simulink subsystem "Controllers"  (R2024b)
settings: Solver=VariableStepAuto  StartTime=0.0  StopTime=10.0  RelTol=1e-3
values from neighbouring files (symbols this model uses):
  CarrierFreq = 150    [init_MMC_HVDC_200.m]
  freq_left = 50    [init_MMC_HVDC_200.m]
  freq_right = 50    [init_MMC_HVDC_200.m]
  Ll = 0.04889    [init_MMC_HVDC_200.m]
  nb_cell = numberOfCell    (= 200)    [init_MMC_HVDC_200.m]
  numberOfCell = 200    [init_MMC_HVDC_200.m]
  P_AC = 1000e6    (= 1000000000)    [init_MMC_HVDC_200.m]
  Rl = 0    [init_MMC_HVDC_200.m]
  Tctrl = Ts    (= 3.5e-05)    [init_MMC_HVDC_200.m]
  Ts = 35e-6    (= 3.5e-05)    [init_MMC_HVDC_200.m]
  V_AC_sec = 320e3    (= 320000)    [init_MMC_HVDC_200.m]
undefined symbols (not defined in the file or in its folder): dend, DiscIntNeverNeededParam, numd
libraries: powerlib_extras x12, simulink x10
(part 1 of 4)
Description:
  | MMC HVDC controllers
settings Model: Creator=Kyle  LastModifiedBy=CD8435

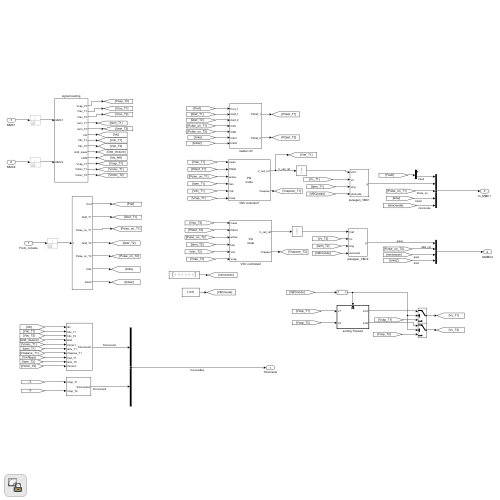
[thumbnail: Simulink's stored preview of the top-level diagram]
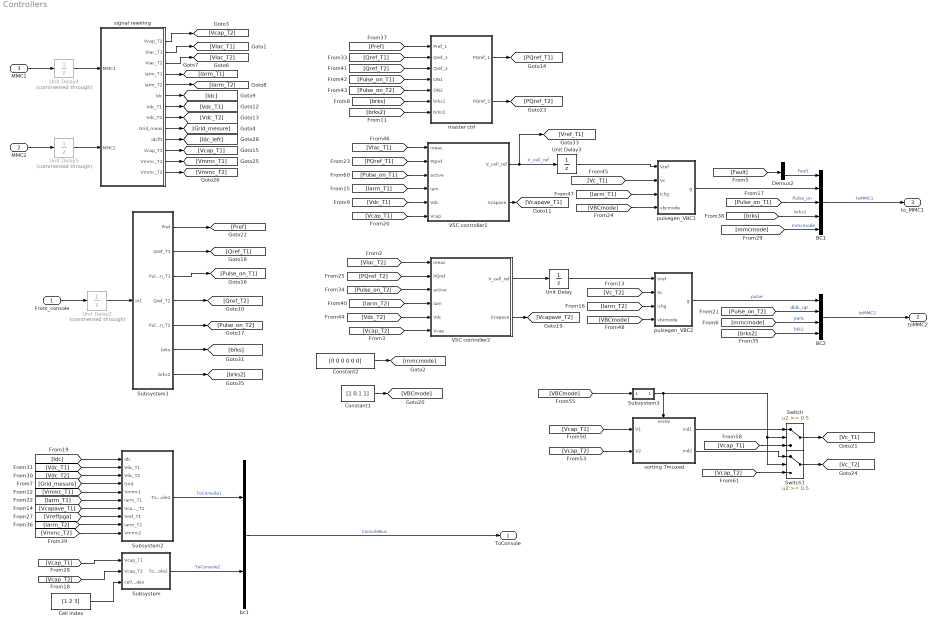
== system Controllers ==
  From_console : Inport
  MMC2 : Inport  Port=2
  MMC1 : Inport  Port=3
  BC1 : BusCreator  Inputs=5  OutDataTypeStr=Bus: toMMC1  NonVirtualBus=on
  BC2 : BusCreator  Inputs=4  OutDataTypeStr=Bus: toMMC2  NonVirtualBus=on
  Cell index : Constant  Value=[1 2 3]
  Constant1 : Constant  Value=[1 0.1 1]
  Constant2 : Constant  Value=[0 0 0 0 0 0]
  Demux2 : Demux  Outputs=2
  Subsystem : Subsystem
  Subsystem1 : Subsystem  mask{brk1=0.15, brk2=0.15, act1=0.25, act2=0.25}
  Subsystem2 : Subsystem
  Subsystem3 : Subsystem
  Switch : Switch  Threshold=0.5  SaturateOnIntegerOverflow=off  InputSameDT=off
  Switch1 : Switch  Threshold=0.5  SaturateOnIntegerOverflow=off  InputSameDT=off
  Unit Delay : UnitDelay  SampleTime=Ts  HasFrameUpgradeWarning=on
  Unit Delay2 : UnitDelay  Commented=through  SampleTime=Ts  HasFrameUpgradeWarning=on
  Unit Delay3 : UnitDelay  SampleTime=Ts  HasFrameUpgradeWarning=on
  Unit Delay4 : UnitDelay  Commented=through  SampleTime=Ts  HasFrameUpgradeWarning=on
  Unit Delay5 : UnitDelay  Commented=through  SampleTime=Ts  HasFrameUpgradeWarning=on
  VSC controller1 : Subsystem  mask(MMC converter controller){cm=off, base=[P_AC, V_AC_sec*1,  E, freq_left], LRx=[Ll, Rl]/2, LRx_inpu=off, Kd=[0.3  2]*10/6  %was [1 0.1]   ; [0.1  1]*1, Kp=[0.3 1]*1     %was [1 0.1]   ; [0.1  1]*1, Kvdc=[0.5*4*1 0.5*2]*1;   %was [0.5 1]*20 for Cdc=320uF, Vabc_lim=[-1 1], limitVdq=1.1, nadv=6, xtrIctrl1=[0.4 10 10 -10], Ts=Tctrl}
      mask prompts: cm "Control mode (check VQ/uncheck PQ), only one terminal in VQ mode"; base "Base value for power(VA), ac voltage(V), dc voltage to ground(V), and frequenvy(Hz) [Sb, Vb, Vdcb,freq]"; LRx "commutation inductance and resistance [Lx, Rx]"; LRx_inpu "[Lx, Rx] in pu if checked/ SI unchecked"; Kd "Kp Ki for d-axis PI control [kp ki]"; Kp "Kp Ki for q-axis PI control [kp ki]"; Kvdc "Kp Ki for Vdc PI control [kp ki]"; Vabc_lim "output Vabc limit [min max]"; limitVdq "Limit for Vd,Vq (pu, default = 1.1)"; nadv "nb of time step to compesate for delay (default=1)"; xtrIctrl1 "[kp, kp, limitmax, limitmin] for current control (default=[0.4, 10, 10, -10])"
      mask init:
      | if cm==0;
      |     x=['PQ\nmode'];
      | else
      |     x=['VQ\nmode'];
      | end
      | 
      | Sb=base(1);            %VA 3phase power base;
      | Vb=base(2);       %V, line-line rms voltage base
      | Ib=Sb/(sqrt(3)*Vb); %A, rms current base
      | Zb=Vb^2/Sb ;        %ohm, impedence base
      | Vdc=base(3);      %V Vdc+ to ground or ground to Vdc- 
      | frq=base(4);
      | 
      | if LRx_inpu
      |     Rxpu=LRx(2);
      |     Lxpu=LRx(1);
      | else
      |     Rxpu=LRx(2)/Zb;
      |     Lxpu=LRx(1)*2*pi*frq/Zb;
      | end;
      | 
      | ks=Vdc*sqrt(3/2)/Vb;     % ma=1/ks for 1pu dc ->1pu ac;
      | 
      | Kp=Kd;
      mask DialogControl ParameterTabVar0 Prompt: Parameters
      mask DialogControl ParameterTabVar01 Prompt: Advanced
      mask Display: disp (x);
  VSC controller2 : Subsystem  mask(MMC converter controller){cm=on, base=[P_AC, V_AC_sec*1,  E, freq_right], LRx=[Ll, Rl]/2, LRx_inpu=off, Kd=[0.3  2]*10/6  %was [1 0.1]   ; [0.1  1]*1, Kp=[0.3 1]*1     %was [1 0.1]   ; [0.1  1]*1, Kvdc=[0.5*4*1 0.5*2]*1;   %was [0.5 1]*20 for Cdc=320uF, Vabc_lim=[-1 1], limitVdq=1.1, nadv=6, xtrIctrl1=[0.4 10 10 -10], Ts=Tctrl}
      mask prompts: cm "Control mode (check VQ/uncheck PQ), only one terminal in VQ mode"; base "Base value for power(VA), ac voltage(V), dc voltage to ground(V), and frequenvy(Hz) [Sb, Vb, Vdcb,freq]"; LRx "commutation inductance and resistance [Lx, Rx]"; LRx_inpu "[Lx, Rx] in pu if checked/ SI unchecked"; Kd "Kp Ki for d-axis PI control [kp ki]"; Kp "Kp Ki for q-axis PI control [kp ki]"; Kvdc "Kp Ki for Vdc PI control [kp ki]"; Vabc_lim "output Vabc limit [min max]"; limitVdq "Limit for Vd,Vq (pu, default = 1.1)"; nadv "nb of time step to compesate for delay (default=1)"; xtrIctrl1 "[kp, kp, limitmax, limitmin] for current control (default=[0.4, 10, 10, -10])"
      mask init: same as Controllers/VSC controller1
      mask DialogControl ParameterTabVar0 Prompt: Parameters
      mask DialogControl ParameterTabVar01 Prompt: Advanced
      mask Display: disp (x);
  bc1 : BusCreator  Inputs=2  OutDataTypeStr=Bus: ConsoleBus  NonVirtualBus=on
  master ctrl : Subsystem
  pulsegen_VBC1 : Subsystem
  pulsegen_VBC2 : Subsystem
  signal rewiring : Subsystem
  sorting Tmuxed : Subsystem
  ToConsole : Outport  VectorParamsAs1DForOutWhenUnconnected=off
  toMMC2 : Outport  Port=2  VectorParamsAs1DForOutWhenUnconnected=off
  to_MMC1 : Outport  Port=3  VectorParamsAs1DForOutWhenUnconnected=off
  wires:
  Subsystem2/1(ToConsole1) -> bc1/1  "ToConsole1"
  From_console/1 -> Unit Delay2/1
  MMC1/1 -> Unit Delay4/1
  MMC2/1 -> Unit Delay5/1
  Subsystem/1(ToConsole2) -> bc1/2  "ToConsole2"
  [Idc] -> Subsystem2/1(Idc)
  [Vdc_T1] -> Subsystem2/2(Vdc_T1)
  [Vdc_T2] -> Subsystem2/3(Vdc_T2)
  [Grid_mesure] -> Subsystem2/4(Grid)
  [Vmmc_T1] -> Subsystem2/5(Vmmc1)
  [Iarm_T1] -> Subsystem2/6(Iarm_T1)
  [Vcapave_T1] -> Subsystem2/7(Vcapave_T1)
  [Vreffpga] -> Subsystem2/8(Vref_T1)
  [Iarm_T2] -> Subsystem2/9(Iarm_T2)
  [Vmmc_T2] -> Subsystem2/10(Vmmc2)
  [Vcap_T1] -> Subsystem/1(Vcap_T1)
  [Vcap_T2] -> Subsystem/2(Vcap_T2)
  signal rewiring/1(Vcap_T2) -> [Vcap_T2]
  signal rewiring/2(VIac_T1) -> [VIac_T1]
  signal rewiring/3(VIac_T2) -> [VIac_T2]
  signal rewiring/4(Iarm_T1) -> [Iarm_T1]
  signal rewiring/5(Iarm_T2) -> [Iarm_T2]
  signal rewiring/9(Grid_meas) -> [Grid_mesure]
  signal rewiring/6(Idc) -> [Idc]
  signal rewiring/7(Vdc_T1) -> [Vdc_T1]
  signal rewiring/8(Vdc_T2) -> [Vdc_T2]
  signal rewiring/10(Idcflt) -> [Idc_left]
  signal rewiring/11(Vcap_T1) -> [Vcap_T1]
  signal rewiring/12(Vmmc_T1) -> [Vmmc_T1]
  signal rewiring/13(Vmmc_T2) -> [Vmmc_T2]
  Subsystem1/2(Qref_T1) -> [Qref_T1]
  Subsystem1/4(Qref_T2) -> [Qref_T2]
  Subsystem1/1(Pref) -> [Pref]
  Subsystem1/6(brks) -> [brks]
  Subsystem1/7(brks2) -> [brks2]
  Subsystem1/5(Pulse_on_T2) -> [Pulse_on_T2]
  Subsystem1/3(Pulse_on_T1) -> [Pulse_on_T1]
  [Vcap_T1] -> sorting Tmuxed/1(V1)
  [Vcap_T2] -> sorting Tmuxed/2(V2)
  sorting Tmuxed/1(ind1) -> Switch/1
  sorting Tmuxed/2(ind2) -> Switch1/1
  [VBCmode] -> Subsystem3/1(In1)
  Subsystem3/1(Out1) -> sorting Tmuxed/Enable, Switch/2, Switch1/2
  Switch/1 -> [Vc_T1]
  [Vcap_T1] -> Switch/3
  Switch1/1 -> [Vc_T2]
  [Vcap_T2] -> Switch1/3
  [Fault] -> Demux2/1
  VSC controller2/1(V_cell_ref) -> Unit Delay/1
  [Pref] -> master ctrl/1(Pref_1)
  [Qref_T1] -> master ctrl/2(Qref_1)
  [Qref_T2] -> master ctrl/3(Qref_2)
  master ctrl/1(PQref_1) -> [PQref_T1]
  master ctrl/2(PQref_2) -> [PQref_T2]
  [Pulse_on_T1] -> master ctrl/4(ON1)
  [Pulse_on_T2] -> master ctrl/5(ON2)
  [Pulse_on_T1] -> VSC controller1/3(active)
  [VIac_T1] -> VSC controller1/1(meas)
  [PQref_T1] -> VSC controller1/2(PQref)
  [Iarm_T1] -> VSC controller1/4(Iam)
  VSC controller1/1(V_cell_ref) -> [Vref_T1], Unit Delay3/1  "V_cell_ref"
  [Pulse_on_T2] -> BC2/2  "dblk_rgt"
  [mmcmode] -> BC2/3  "para"
  [brks2] -> BC2/4  "brk2"
  [Vdc_T1] -> VSC controller1/5(Vdc)
  [Vcap_T1] -> VSC controller1/6(Vcap)
  VSC controller1/2(Vcapave) -> [Vcapave_T1]
  [VIac_T2] -> VSC controller2/1(meas)
  [PQref_T2] -> VSC controller2/2(PQref)
  [Pulse_on_T2] -> VSC controller2/3(active)
  [Iarm_T2] -> VSC controller2/4(Iam)
  [Vdc_T2] -> VSC controller2/5(Vdc)
  [Vcap_T2] -> VSC controller2/6(Vcap)
  VSC controller2/2(Vcapave) -> [Vcapave_T2]
  [brks] -> master ctrl/6(brks1)
  [brks2] -> master ctrl/7(brks2)
  pulsegen_VBC2/1(g) -> BC2/1  "pulse"
  [Pulse_on_T1] -> BC1/3  "Pulse_on"
  [brks] -> BC1/4  "brks2"
  Demux2/2 -> BC1/1  "Fault"
  [mmcmode] -> BC1/5  "mmcmode"
  [Vc_T1] -> pulsegen_VBC1/2(Vc)
  [Iarm_T1] -> pulsegen_VBC1/3(ichg)
  pulsegen_VBC1/1(g) -> BC1/2
  [VBCmode] -> pulsegen_VBC1/4(vbcmode)
  [Vc_T2] -> pulsegen_VBC2/2(Vc)
  [Iarm_T2] -> pulsegen_VBC2/3(ichg)
  [VBCmode] -> pulsegen_VBC2/4(vbcmode)
  Constant1/1 -> [VBCmode]
  Constant2/1 -> [mmcmode]
  Unit Delay/1 -> pulsegen_VBC2/1(Vref)
  Unit Delay3/1 -> pulsegen_VBC1/1(Vref)
  Unit Delay4/1 -> signal rewiring/1(MMC1)
  Unit Delay5/1 -> signal rewiring/2(MMC2)
  Unit Delay2/1 -> Subsystem1/1(In1)
  BC1/1 -> to_MMC1/1  "toMMC1"
  BC2/1 -> toMMC2/1  "toMMC2"
  bc1/1 -> ToConsole/1  "ConsoleBus"
  Cell index/1 -> Subsystem/3(cellindex)

== system Controllers/Subsystem ==
  Vcap_T1 : Inport
  Vcap_T2 : Inport  Port=2
  cellindex : Inport  Port=3
  Bus Creator : BusCreator  Inputs=2
  Subsystem1 : Subsystem
  Subsystem3 : Subsystem
  ToConsole2 : Outport  VectorParamsAs1DForOutWhenUnconnected=off
  wires:
  cellindex/1 -> Subsystem1/2(CellIndex)
  Vcap_T2/1 -> Subsystem3/1(In1)
  Vcap_T1/1 -> Subsystem1/1(In1)
  Bus Creator/1 -> ToConsole2/1
  Subsystem1/1(Out1) -> Bus Creator/1  "Vcap_T1"
  Subsystem3/1(Out1) -> Bus Creator/2  "Vcap_T2"

== system Controllers/Subsystem1 ==
  In1 : Inport
  Bus Selector : BusSelector  OutputSignals=PQref.Pref,PQref.Qref_T1,PQref.Pulse_on_T1,Q2.signal1,Q2.Pulse_on_T2,breakers.dcbrk,breakers.ac_brk_T1,breakers.ac_brk_T2
  Mux5 : Mux  Inputs=2
  Product{,1..3} (4 alike) : Product  RndMeth=Zero
  Step : Step  Time=brk1  SampleTime=Ts
  Step1 : Step  Time=brk2  SampleTime=Ts
  Step2 : Step  Time=act2  SampleTime=Ts
  Step3 : Step  Time=act1  SampleTime=Ts
  Pref : Outport  VectorParamsAs1DForOutWhenUnconnected=off
  Qref_T1 : Outport  Port=2  VectorParamsAs1DForOutWhenUnconnected=off
  Pulse_on_T1 : Outport  Port=3  VectorParamsAs1DForOutWhenUnconnected=off
  Qref_T2 : Outport  Port=4  VectorParamsAs1DForOutWhenUnconnected=off
  Pulse_on_T2 : Outport  Port=5  VectorParamsAs1DForOutWhenUnconnected=off
  brks : Outport  Port=6  VectorParamsAs1DForOutWhenUnconnected=off
  brks2 : Outport  Port=7  VectorParamsAs1DForOutWhenUnconnected=off
  wires:
  Step/1 -> Product/2
  Step1/1 -> Product1/2
  Step2/1 -> Product2/2
  Bus Selector/5 -> Product2/1  "<Pulse_on_T2>"
  Bus Selector/3 -> Product3/1  "<Pulse_on_T1>"
  Step3/1 -> Product3/2
  Bus Selector/2 -> Qref_T1/1  "<Qref_T1>"
  Product3/1 -> Pulse_on_T1/1
  Bus Selector/4 -> Qref_T2/1  "<signal1>"
  In1/1 -> Bus Selector/1
  Product2/1 -> Pulse_on_T2/1
  Product/1 -> brks/1
  Product1/1 -> brks2/1
  Mux5/1 -> Product/1
  Bus Selector/1 -> Pref/1  "<Pref>"
  Bus Selector/6 -> Mux5/1  "<dcbrk>"
  Bus Selector/7 -> Mux5/2  "<ac_brk_T1>"
  Bus Selector/8 -> Product1/1  "<ac_brk_T2>"

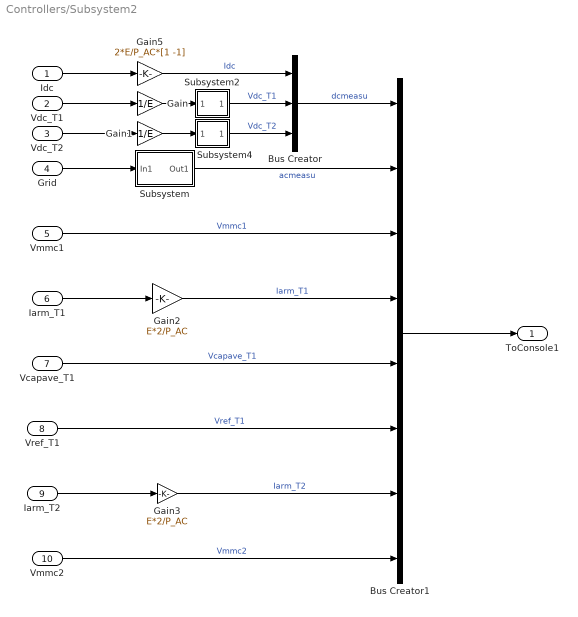
== system Controllers/Subsystem2 ==
  Idc : Inport
  Vdc_T1 : Inport  Port=2
  Vdc_T2 : Inport  Port=3
  Grid : Inport  Port=4
  Vmmc1 : Inport  Port=5
  Iarm_T1 : Inport  Port=6
  Vcapave_T1 : Inport  Port=7
  Vref_T1 : Inport  Port=8
  Iarm_T2 : Inport  Port=9
  Vmmc2 : Inport  Port=10
  Bus Creator : BusCreator  Inputs=3
  Bus Creator1 : BusCreator  Inputs=8
  Gain : Gain  Gain=1/E
  Gain1 : Gain  Gain=1/E
  Gain2 : Gain  Gain=E*2/P_AC
  Gain3 : Gain  Gain=E*2/P_AC
  Gain5 : Gain  Gain=2*E/P_AC*[1 -1]
  Subsystem : Subsystem
  Subsystem2 : Subsystem
  Subsystem4 : Subsystem
  ToConsole1 : Outport  VectorParamsAs1DForOutWhenUnconnected=off
  wires:
  Subsystem4/1(Out1) -> Bus Creator/3  "Vdc_T2"
  Subsystem2/1(Out1) -> Bus Creator/2  "Vdc_T1"
  Gain3/1 -> Bus Creator1/7  "Iarm_T2"
  Iarm_T2/1 -> Gain3/1
  Vmmc2/1 -> Bus Creator1/8  "Vmmc2"
  Vref_T1/1 -> Bus Creator1/6  "Vref_T1"
  Vcapave_T1/1 -> Bus Creator1/5  "Vcapave_T1"
  Vmmc1/1 -> Bus Creator1/3  "Vmmc1"
  Iarm_T1/1 -> Gain2/1
  Vdc_T2/1 -> Gain1/1
  Vdc_T1/1 -> Gain/1
  Grid/1 -> Subsystem/1(In1)
  Bus Creator1/1 -> ToConsole1/1
  Gain2/1 -> Bus Creator1/4  "Iarm_T1"
  Subsystem/1(Out1) -> Bus Creator1/2  "acmeasu"
  Gain1/1 -> Subsystem4/1(In1)
  Gain/1 -> Subsystem2/1(In1)
  Gain5/1 -> Bus Creator/1  "Idc"
  Idc/1 -> Gain5/1
  Bus Creator/1 -> Bus Creator1/1  "dcmeasu"

== system Controllers/Subsystem3 ==
  In1 : Inport
  Compare To Constant1 : simulink/Logic and Bit Operations/Compare To Constant  relop===  const=2  OutDataTypeStr=uint8
  Compare To Constant2 : simulink/Logic and Bit Operations/Compare To Constant  relop===  const=12  OutDataTypeStr=uint8
  Demux1 : Demux  Outputs=[1 -1]
  Logical Operator : Logic  Operator=OR  AllPortsSameDT=off  OutDataTypeStr=boolean
  Out1 : Outport  VectorParamsAs1DForOutWhenUnconnected=off
  wires:
  Logical Operator/1 -> Out1/1
  Demux1/1 -> Compare To Constant1/1, Compare To Constant2/1
  Compare To Constant2/1 -> Logical Operator/2
  Compare To Constant1/1 -> Logical Operator/1
  In1/1 -> Demux1/1

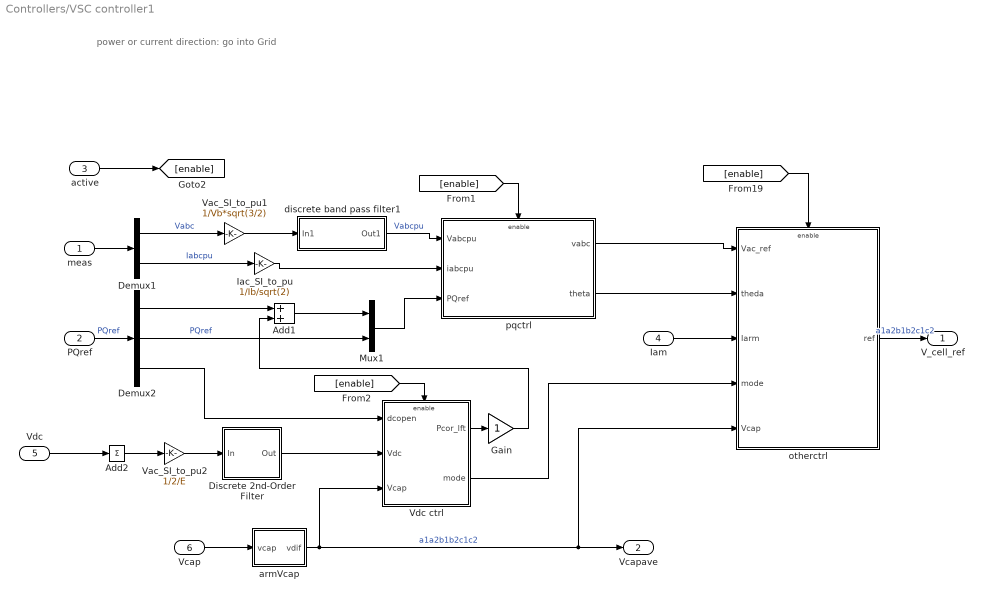
== system Controllers/VSC controller1 ==
  note: power or current direction: go into Grid
  meas : Inport
  PQref : Inport  Port=2
  active : Inport  Port=3
  Iam : Inport  Port=4
  Vdc : Inport  Port=5
  Vcap : Inport  Port=6
  Add1 : Sum
  Add2 : Sum  Inputs=1
  Demux1 : Demux  Outputs=[3 3 ]
  Demux2 : Demux  Outputs=3
  Discrete 2nd-Order Filter : Subsystem  mask(Discrete 2nd-Order Filter){FilterType=Lowpass, Fo=90, Zeta=0.707, Ts=Ts, Initialize=off, Vac_Init=[0.8 -25 60], Vdc_Init=-0.4, PlotResponse=off, param1=[1 500 1]}
      mask prompts: FilterType "Filter Type:"; Fo "Cut-off frequency (Hz):"; Zeta "Damping factor Zeta ( Q = 1 / (2*Zeta) ):"; Ts "Sample time:"; Initialize "Initialize filter states"; Vac_Init "AC initial input: [ Mag  Phase(degrees)  Freq(Hz) ]"; Vdc_Init "DC Initial input:"; PlotResponse "Plot filter response"; param1 "Frequency range(Hz) : [Start  End  Inc.]"
      mask init:
      | str=sprintf(' Fo=%iHz\n\n',Fo);
      | Wo=2*pi*Fo;
      | switch FilterType
      | case 1, % Lowpass
      |        X=[0 1 2 3 4];
      |        Y=[-2 -2 -3 -4 -4];
      |        n2=0;n1=0;n0=Wo*Wo;
      |        d2=1;d1=2*Zeta*Wo;d0=Wo*Wo;
      | 	   Ystep=1;
      |  case 2,   % Highpass
      |        X=[0 1 2 3 4];
      |        Y=[-4 -4 -3 -2 -2];
      |        n2=1;n1=0;n0=0;
      |        d2=1;d1=2*Zeta*Wo;d0=Wo*Wo;
      | 	   Ystep=2;
      |     case 3,   % Bandpass
      |        X=[0 1 2 3 4 5 ];
      |        Y=[-3 -3 -2 -2 -3 -3];
      |        n2=0;n1=2*Zeta*Wo;n0=0;
      |        d2=1;d1=2*Zeta*Wo;d0=Wo*Wo;
      | 	   Ystep=3;
      |     case 4,  %Bandstop (Notch)
      |        X=[0 1 2 3 4 5 ];
      |        Y=[-2 -2 -3 -3 -2 -2];
      |        n2=1;n1=0;n0=Wo*Wo;
      |        d2=1;d1=2*Zeta*Wo;d0=Wo*Wo;
      | 	   Ystep=4;
      |     end
      | %
      | numc=[n2 n1 n0];
      | denc=[d2 d1 d0];
      | [Ac,Bc,Cc,Dc]=tf2ss(numc,denc);
      | %
      | %  Conversion to discrete transfer function
      | nstates = size(Ac,1);
      | invexp = inv(eye(nstates) - (Ts/2)*Ac);
      | Ad = invexp*(eye(nstates) + (Ts/2)*Ac);
      | Bd = invexp*Bc;
      | Cd = Cc*invexp*Ts;
      | Dd = Cc*invexp*Bc*(Ts/2) + Dc;
      | %
      | if Initialize==1  % Compute initial conditions on states
      | u1=Vac_Init(1)*exp(j*Vac_Init(2)*pi/180);
      | u2=Vdc_Init*exp(j*90*pi/180);
      | u=u1+u2;
      | u0=imag(u); % input at  t=0;
      | I=eye(size(Ac));
      | sI1=I*j*(2*pi*Vac_Init(3));
      | sI2=I*j*0;
      | x=inv(sI1-Ac)*Bc*u1 + inv(sI2-Ac)*Bc*u2;
      | x0c=imag(x);
      | x0d=(I-Ac*Ts/2)*x0c/Ts - Bc/2*u0;
      | else
      | x0d=0;
      | end
      | %
      | if PlotResponse==1 % Plot frequency and step response
      | if Zeta==1
      | 	z=1+1e-12;
      | else
      | 	z=Zeta;
      | end
      | wn=Wo;
      | t=[0:1/(z*wn)/1000:7/(z*wn)];
      | f=param1(1):param1(3):param1(2);
      | w=2*pi*f;
      | switch FilterType
      | 	case 1, % Lowpass
      | 		Ystep=wn^2*(1/wn^2+1/(4*z^2*wn^2-4*wn^2)^(1/2)*(1/(-z*wn+1/2*(4*z^2*wn^2-4*wn^2)^(1/2))*exp((-z*wn+1/2*(4*z^2*wn^2-4*wn^2)^(1/2))*t)-1/(-z*wn-1/2*(4*z^2*wn^2-4*wn^2)^(1/2))*exp((-z*wn-1/2*(4*z^2*wn^2-4*wn^2)^(1/2))*t)));
      | 		numFreq=wn^2;
      | 	case 2,   % Highpass
      | 		Ystep=-exp(-z*wn*t)/(z-1)/(z+1).*cos((-wn^2*(z-1)*(z+1))^(1/2)*t)+exp(-z*wn*t)/(z-1)/(z+1)*z^2.*cos((-wn^2*(z-1)*(z+1))^(1/2)*t)+z/wn*exp(-z*wn*t)/(z-1)/(z+1)*(wn^2-z^2*wn^2)^(1/2).*sin((-wn^2*(z-1)*(z+1))^(1/2)*t);
      | 		numFreq=-w.^2;
      | 	case 3,   % Bandpass
      | 		Ystep=2*z*wn/(4*z^2*wn^2-4*wn^2)^(1/2)*(exp((-z*wn+1/2*(4*z^2*wn^2-4*wn^2)^(1/2))*t)-exp((-z*wn-1/2*(4*z^2*wn^2-4*wn^2)^(1/2))*t));
      | 		numFreq=2*Zeta*wn.*w*j;
      | 	case 4,  %Bandstop (Notch)
      | 		Ystep=1+2*z/wn*exp(-z*wn*t)/(z-1)/(z+1)*(wn^2-z^2*wn^2)^(1/2).*sin((-wn^2*(z-1)*(z+1))^(1/2)*t);	
      | 		numFreq=wn^2-w.^2;
      | end
      | %
      | denFreq=(wn^2-w.^2) + 2*Zeta*wn*j.*w;
      | RepFreq=numFreq./denFreq;
      | Mag=abs(RepFreq);
      | Pha=angle(RepFreq)*180/pi;
      | %
      | figure(1)
      | subplot(2,1,1)
      | plot(f,Mag)
      | grid
      | title('Bode Diagram')
      | ylabel('Magnitude')
      | subplot(2,1,2)
      | plot(f,Pha)
      | ylabel('Phase (deg)')
      | xlabel('Frequency (Hz)')
      | grid
      | figure(2)
      | plot(t,real(Ystep))
      | grid
      | ylabel('Amplitude')
      | xlabel('Time (s)')
      | title('Step Response')
      | end
      | power_initmask();
      mask Help: This block is part of a subset of blocks in the Extras library that does not have documentation associated with it, other than the block mask description.
      mask TypeOptions FilterType: Lowpass | Highpass | Bandpass | Bandstop (Notch)
      mask Callback Initialize: p5=get_param(gcb,'Initialize');if strcmp(p5,'on');visible={'on','on','on','on','on','on','on','on',get_param(gcb,'PlotResponse')};else;visible={'on','on','on','on','on','off','off','on',get_param(gcb,'PlotResponse')};end;set_param(gcb,'MaskVisibilities',visible)
      mask Callback PlotResponse: p8=get_param(gcb,'PlotResponse');if strcmp(p8,'on');visible={'on','on','on','on','on',get_param(gcb,'Initialize'),get_param(gcb,'Initialize'),'on','on'};else;visible={'on','on','on','on','on',get_param(gcb,'Initialize'),get_param(gcb,'Initialize'),'on','off'};end;set_param(gcb,'MaskVisibilities',visible)
      mask Display:
      | plot(X,Y);
      | disp(str);
  Gain : Gain
  Iac_SI_to_pu : Gain  Gain=1/Ib/sqrt(2)
  Mux1 : Mux  Inputs=2
  Vac_SI_to_pu1 : Gain  Gain=1/Vb*sqrt(3/2)
  Vac_SI_to_pu2 : Gain  Gain=1/2/E  SampleTime=Tctrl
  Vdc ctrl : Subsystem
  armVcap : Subsystem
  discrete band pass filter1 : Subsystem  mask(discrete transfer Fcn generator){Fo=frq, adj1=1, inistate=0, Ts=Ts, bodedw=off}
      mask prompts: Fo "F0 (Hz)"; adj1 "adj (1 for no adjustment, larger adj for wider band pass)"; inistate "Initial states"; Ts "Sample time (must be explicite)"; bodedw "draw Bode diagram of filter"
      mask help:
      | This block transfer a continous TF to a discrete TF
      | using Bilinear (Tustin) approximation
      mask init:
      | AD1=tf([1 0],1);
      | 
      | %second order
      | % Fo=50; %cut off freq.
      | % omega0=Fo*2*pi;
      | % adj1=3;   %adjustment 1
      | Zeta= 0.707*adj1; %Damping factor Zeta ( Q = 1 / (2*Zeta) ):
      | Wo=2*pi*Fo;
      | % str=sprintf(' Fo=%iHz\n\n',Fo);
      |  n2=0; n1=0;n0=Wo*Wo;
      |  d2=1;d1=2*Zeta*Wo;d0=Wo*Wo;
      | numc=[n2 n1 n0];
      | denc=[d2 d1 d0];
      | AD3=tf(numc,denc);
      | 
      | AD4=AD1*AD3;
      | [mag1,pha1]=bode(AD4,Wo);
      | mag0=mag1;
      | AD=AD4/mag0;
      | 
      | if bodedw==1
      |     figure;
      |     h=bodeplot(AD1,AD3,AD);
      |     setoptions(h,'FreqUnits','Hz');
      |     grid on;
      |     title(['Bode Diagram, adj=',num2str(adj1)]);
      | end;
      |     
      | % gg=tf(num,den);
      | ggd=c2d(AD,Ts,'tustin');
      | [numd,dend] = tfdata(ggd,'v');
  otherctrl : Subsystem
  pqctrl : Subsystem
  V_cell_ref : Outport  VectorParamsAs1DForOutWhenUnconnected=off
  Vcapave : Outport  Port=2  VectorParamsAs1DForOutWhenUnconnected=off
  wires:
  otherctrl/1(ref) -> V_cell_ref/1  "a1a2b1b2c1c2"
  pqctrl/2(theta) -> otherctrl/2(theda)
  pqctrl/1(vabc) -> otherctrl/1(Vac_ref)
  PQref/1 -> Demux2/1  "PQref"
  active/1 -> [enable]
  Iam/1 -> otherctrl/3(Iarm)
  discrete band pass filter1/1(Out1) -> pqctrl/1(Vabcpu)  "Vabcpu"
  meas/1 -> Demux1/1
  Demux1/2 -> Iac_SI_to_pu/1  "Iabcpu"
  Demux1/1 -> Vac_SI_to_pu1/1  "Vabc"
  Iac_SI_to_pu/1 -> pqctrl/2(iabcpu)
  Vdc/1 -> Add2/1
  Vcap/1 -> armVcap/1(vcap)
  armVcap/1(vdif) -> Vdc ctrl/3(Vcap), Vcapave/1, otherctrl/5(Vcap)  "a1a2b1b2c1c2"
  Vdc ctrl/2(mode) -> otherctrl/4(mode)
  Demux2/1 -> Add1/1
  Vdc ctrl/1(Pcor_lft) -> Gain/1
  Add1/1 -> Mux1/1
  Demux2/2 -> Mux1/2  "PQref"
  Mux1/1 -> pqctrl/3(PQref)
  Discrete 2nd-Order Filter/1(Out) -> Vdc ctrl/2(Vdc)
  Add2/1 -> Vac_SI_to_pu2/1
  Vac_SI_to_pu2/1 -> Discrete 2nd-Order Filter/1(In)
  Gain/1 -> Add1/2
  Vac_SI_to_pu1/1 -> discrete band pass filter1/1(In1)
  Demux2/3 -> Vdc ctrl/1(dcopen)
  [enable] -> otherctrl/Enable
  [enable] -> pqctrl/Enable
  [enable] -> Vdc ctrl/Enable

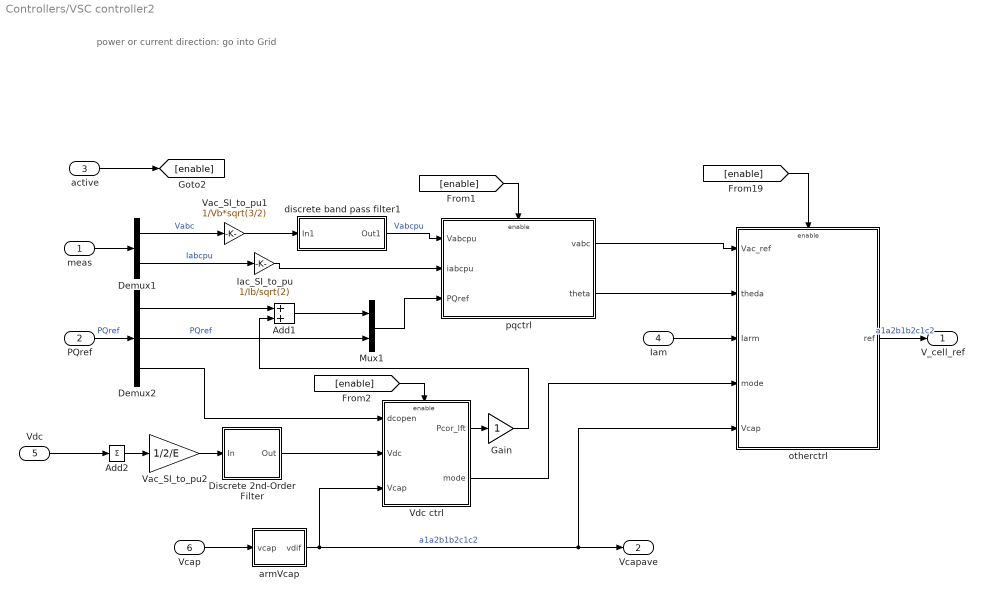
== system Controllers/VSC controller2 ==
  note: power or current direction: go into Grid
  meas : Inport
  PQref : Inport  Port=2
  active : Inport  Port=3
  Iam : Inport  Port=4
  Vdc : Inport  Port=5
  Vcap : Inport  Port=6
  Add1 : Sum
  Add2 : Sum  Inputs=1
  Demux1 : Demux  Outputs=[3 3 ]
  Demux2 : Demux  Outputs=3
  Discrete 2nd-Order Filter : Subsystem  mask(Discrete 2nd-Order Filter){FilterType=Lowpass, Fo=90, Zeta=0.707, Ts=Ts, Initialize=off, Vac_Init=[0.8 -25 60], Vdc_Init=-0.4, PlotResponse=off, param1=[1 500 1]}
      mask prompts: FilterType "Filter Type:"; Fo "Cut-off frequency (Hz):"; Zeta "Damping factor Zeta ( Q = 1 / (2*Zeta) ):"; Ts "Sample time:"; Initialize "Initialize filter states"; Vac_Init "AC initial input: [ Mag  Phase(degrees)  Freq(Hz) ]"; Vdc_Init "DC Initial input:"; PlotResponse "Plot filter response"; param1 "Frequency range(Hz) : [Start  End  Inc.]"
      mask init: same as Controllers/VSC controller1/Discrete 2nd-Order Filter
      mask Help: This block is part of a subset of blocks in the Extras library that does not have documentation associated with it, other than the block mask description.
      mask TypeOptions FilterType: Lowpass | Highpass | Bandpass | Bandstop (Notch)
      mask Callback Initialize: p5=get_param(gcb,'Initialize');if strcmp(p5,'on');visible={'on','on','on','on','on','on','on','on',get_param(gcb,'PlotResponse')};else;visible={'on','on','on','on','on','off','off','on',get_param(gcb,'PlotResponse')};end;set_param(gcb,'MaskVisibilities',visible)
      mask Callback PlotResponse: p8=get_param(gcb,'PlotResponse');if strcmp(p8,'on');visible={'on','on','on','on','on',get_param(gcb,'Initialize'),get_param(gcb,'Initialize'),'on','on'};else;visible={'on','on','on','on','on',get_param(gcb,'Initialize'),get_param(gcb,'Initialize'),'on','off'};end;set_param(gcb,'MaskVisibilities',visible)
      mask Display:
      | plot(X,Y);
      | disp(str);
  Gain : Gain
  Iac_SI_to_pu : Gain  Gain=1/Ib/sqrt(2)
  Mux1 : Mux  Inputs=2
  Vac_SI_to_pu1 : Gain  Gain=1/Vb*sqrt(3/2)
  Vac_SI_to_pu2 : Gain  Gain=1/2/E  SampleTime=Tctrl
  Vdc ctrl : Subsystem
  armVcap : Subsystem
  discrete band pass filter1 : Subsystem  mask(discrete transfer Fcn generator){Fo=frq, adj1=1, inistate=0, Ts=Ts, bodedw=off}
      mask prompts: Fo "F0 (Hz)"; adj1 "adj (1 for no adjustment, larger adj for wider band pass)"; inistate "Initial states"; Ts "Sample time (must be explicite)"; bodedw "draw Bode diagram of filter"
      mask help:
      | This block transfer a continous TF to a discrete TF
      | using Bilinear (Tustin) approximation
      mask init: same as Controllers/VSC controller1/discrete band pass filter1
  otherctrl : Subsystem
  pqctrl : Subsystem
  V_cell_ref : Outport  VectorParamsAs1DForOutWhenUnconnected=off
  Vcapave : Outport  Port=2  VectorParamsAs1DForOutWhenUnconnected=off
  wires:
  [enable] -> Vdc ctrl/Enable
  [enable] -> pqctrl/Enable
  [enable] -> otherctrl/Enable
  Demux2/3 -> Vdc ctrl/1(dcopen)
  Vac_SI_to_pu1/1 -> discrete band pass filter1/1(In1)
  Gain/1 -> Add1/2
  Vac_SI_to_pu2/1 -> Discrete 2nd-Order Filter/1(In)
  Add2/1 -> Vac_SI_to_pu2/1
  Discrete 2nd-Order Filter/1(Out) -> Vdc ctrl/2(Vdc)
  Mux1/1 -> pqctrl/3(PQref)
  Demux2/2 -> Mux1/2  "PQref"
  Add1/1 -> Mux1/1
  Vdc ctrl/1(Pcor_lft) -> Gain/1
  Demux2/1 -> Add1/1
  Vdc ctrl/2(mode) -> otherctrl/4(mode)
  armVcap/1(vdif) -> otherctrl/5(Vcap), Vcapave/1, Vdc ctrl/3(Vcap)  "a1a2b1b2c1c2"
  Vcap/1 -> armVcap/1(vcap)
  Vdc/1 -> Add2/1
  Iac_SI_to_pu/1 -> pqctrl/2(iabcpu)
  Demux1/1 -> Vac_SI_to_pu1/1  "Vabc"
  Demux1/2 -> Iac_SI_to_pu/1  "Iabcpu"
  meas/1 -> Demux1/1
  discrete band pass filter1/1(Out1) -> pqctrl/1(Vabcpu)  "Vabcpu"
  Iam/1 -> otherctrl/3(Iarm)
  active/1 -> [enable]
  PQref/1 -> Demux2/1  "PQref"
  pqctrl/1(vabc) -> otherctrl/1(Vac_ref)
  pqctrl/2(theta) -> otherctrl/2(theda)
  otherctrl/1(ref) -> V_cell_ref/1  "a1a2b1b2c1c2"

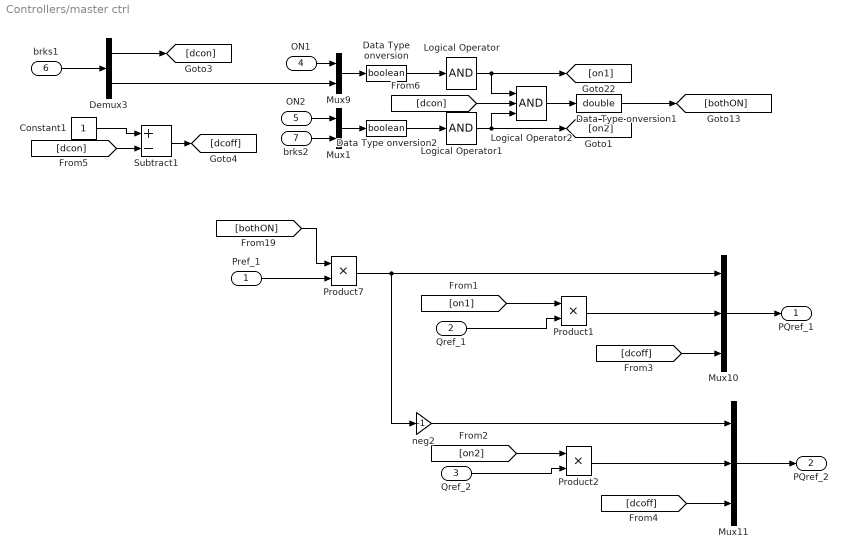
== system Controllers/master ctrl ==
  Pref_1 : Inport
  Qref_1 : Inport  Port=2
  Qref_2 : Inport  Port=3
  ON1 : Inport  Port=4
  ON2 : Inport  Port=5
  brks1 : Inport  Port=6
  brks2 : Inport  Port=7
  Constant1 : Constant
  Data Type onversion : DataTypeConversion  OutDataTypeStr=boolean  SaturateOnIntegerOverflow=off  RndMeth=Floor
  Data Type onversion1 : DataTypeConversion  OutDataTypeStr=double  SaturateOnIntegerOverflow=off  RndMeth=Floor
  Data Type onversion2 : DataTypeConversion  OutDataTypeStr=boolean  SaturateOnIntegerOverflow=off  RndMeth=Floor
  Demux3 : Demux  Outputs=2
  Logical Operator : Logic  Inputs=1  AllPortsSameDT=off  OutDataTypeStr=boolean
  Logical Operator1 : Logic  Inputs=1  AllPortsSameDT=off  OutDataTypeStr=boolean
  Logical Operator2 : Logic  Inputs=3  AllPortsSameDT=off  OutDataTypeStr=boolean
  Mux1 : Mux  Inputs=2
  Mux10 : Mux  Inputs=3
  Mux11 : Mux  Inputs=3
  Mux9 : Mux  Inputs=2
  Product1 : Product  RndMeth=Zero
  Product2 : Product  RndMeth=Zero
  Product7 : Product  RndMeth=Zero
  Subtract1 : Sum  Inputs=+-
  neg2 : Gain  Gain=-1  SampleTime=Tctrl
  PQref_1 : Outport  VectorParamsAs1DForOutWhenUnconnected=off
  PQref_2 : Outport  Port=2  VectorParamsAs1DForOutWhenUnconnected=off
  wires:
  Mux9/1 -> Data Type onversion/1
  Data Type onversion/1 -> Logical Operator/1
  Product1/1 -> Mux10/2
  Product2/1 -> Mux11/2
  Product7/1 -> Mux10/1, neg2/1
  ON1/1 -> Mux9/1
  Mux10/1 -> PQref_1/1
  ON2/1 -> Mux1/1
  Qref_1/1 -> Product1/2
  Mux11/1 -> PQref_2/1
  Qref_2/1 -> Product2/2
  Data Type onversion1/1 -> [bothON]
  [on1] -> Product1/1
  [on2] -> Product2/1
  [bothON] -> Product7/1
  neg2/1 -> Mux11/1
  Pref_1/1 -> Product7/2
  brks1/1 -> Demux3/1
  Demux3/1 -> [dcon]
  Demux3/2 -> Mux9/2
  Logical Operator/1 -> [on1], Logical Operator2/1
  brks2/1 -> Mux1/2
  Data Type onversion2/1 -> Logical Operator1/1
  Mux1/1 -> Data Type onversion2/1
  Logical Operator1/1 -> [on2], Logical Operator2/3
  Logical Operator2/1 -> Data Type onversion1/1
  [dcoff] -> Mux10/3
  [dcoff] -> Mux11/3
  Subtract1/1 -> [dcoff]
  Constant1/1 -> Subtract1/1
  [dcon] -> Subtract1/2
  [dcon] -> Logical Operator2/2

== system Controllers/pulsegen_VBC1 ==
  Vref : Inport
  Vc : Inport  Port=2
  ichg : Inport  Port=3
  vbcmode : Inport  Port=4
  Demux3 : Demux  Outputs=[2 1]
  VBC : Subsystem
  pulse_gen : Subsystem
  g : Outport  VectorParamsAs1DForOutWhenUnconnected=off
  wires:
  pulse_gen/1(A_pulse) -> VBC/1(g)  "pulse"
  pulse_gen/2(NLC) -> VBC/2(NL)
  Vref/1 -> pulse_gen/1(Vcell_ref)
  Vc/1 -> VBC/3(Vc)
  VBC/1(go) -> g/1  "Pulse"
  ichg/1 -> VBC/4(ichg)
  Demux3/1 -> VBC/5(mode)
  vbcmode/1 -> Demux3/1
  Demux3/2 -> pulse_gen/2(pgmode)

== system Controllers/pulsegen_VBC2 ==
  Vref : Inport
  Vc : Inport  Port=2
  ichg : Inport  Port=3
  vbcmode : Inport  Port=4
  Demux3 : Demux  Outputs=[2 1]
  VBC : Subsystem
  pulse_gen : Subsystem
  g : Outport  VectorParamsAs1DForOutWhenUnconnected=off
  wires:
  Demux3/2 -> pulse_gen/2(pgmode)
  vbcmode/1 -> Demux3/1
  Demux3/1 -> VBC/5(mode)
  ichg/1 -> VBC/4(ichg)
  VBC/1(go) -> g/1  "Pulse"
  Vc/1 -> VBC/3(Vc)
  Vref/1 -> pulse_gen/1(Vcell_ref)
  pulse_gen/2(NLC) -> VBC/2(NL)
  pulse_gen/1(A_pulse) -> VBC/1(g)  "pulse"

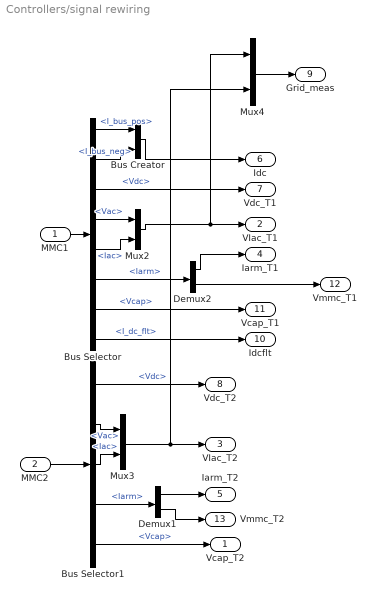
== system Controllers/signal rewiring ==
  MMC1 : Inport
  MMC2 : Inport  Port=2
  Bus Creator : BusCreator  Inputs=2
  Bus Selector : BusSelector  OutputSignals=I_bus_pos,I_bus_neg,VImeas_T1.Vdc,VImeas_T1.Vac,VImeas_T1.Iac,VImeas_T1.Iarm,VImeas_T1.Vcap,I_dc_flt
  Bus Selector1 : BusSelector  OutputSignals=VImeas_T1.Vdc,VImeas_T1.Vac,VImeas_T1.Iac,VImeas_T1.Iarm,VImeas_T1.Vcap
  Demux1 : Demux  Outputs=[6 6]
  Demux2 : Demux  Outputs=[6 6]
  Mux2 : Mux  Inputs=2
  Mux3 : Mux  Inputs=2
  Mux4 : Mux  Inputs=2
  Vcap_T2 : Outport  VectorParamsAs1DForOutWhenUnconnected=off
  VIac_T1 : Outport  Port=2  VectorParamsAs1DForOutWhenUnconnected=off
  VIac_T2 : Outport  Port=3  VectorParamsAs1DForOutWhenUnconnected=off
  Iarm_T1 : Outport  Port=4  VectorParamsAs1DForOutWhenUnconnected=off
  Iarm_T2 : Outport  Port=5  VectorParamsAs1DForOutWhenUnconnected=off
  Idc : Outport  Port=6  VectorParamsAs1DForOutWhenUnconnected=off
  Vdc_T1 : Outport  Port=7  VectorParamsAs1DForOutWhenUnconnected=off
  Vdc_T2 : Outport  Port=8  VectorParamsAs1DForOutWhenUnconnected=off
  Grid_meas : Outport  Port=9  VectorParamsAs1DForOutWhenUnconnected=off
  Idcflt : Outport  Port=10  VectorParamsAs1DForOutWhenUnconnected=off
  Vcap_T1 : Outport  Port=11  VectorParamsAs1DForOutWhenUnconnected=off
  Vmmc_T1 : Outport  Port=12  VectorParamsAs1DForOutWhenUnconnected=off
  Vmmc_T2 : Outport  Port=13  VectorParamsAs1DForOutWhenUnconnected=off
  wires:
  MMC1/1 -> Bus Selector/1
  Bus Creator/1 -> Idc/1
  Bus Selector/3 -> Vdc_T1/1  "<Vdc>"
  Mux2/1 -> VIac_T1/1, Mux4/1
  Bus Selector1/1 -> Vdc_T2/1  "<Vdc>"
  MMC2/1 -> Bus Selector1/1
  Mux4/1 -> Grid_meas/1
  Bus Selector/8 -> Idcflt/1  "<I_dc_flt>"
  Bus Selector1/5 -> Vcap_T2/1  "<Vcap>"
  Bus Selector/7 -> Vcap_T1/1  "<Vcap>"
  Bus Selector/1 -> Bus Creator/1  "<I_bus_pos>"
  Bus Selector/2 -> Bus Creator/2  "<I_bus_neg>"
  Bus Selector/4 -> Mux2/1  "<Vac>"
  Bus Selector/5 -> Mux2/2  "<Iac>"
  Mux3/1 -> VIac_T2/1, Mux4/2
  Bus Selector1/2 -> Mux3/1  "<Vac>"
  Bus Selector1/3 -> Mux3/2  "<Iac>"
  Bus Selector/6 -> Demux2/1  "<Iarm>"
  Demux2/1 -> Iarm_T1/1
  Demux2/2 -> Vmmc_T1/1
  Bus Selector1/4 -> Demux1/1  "<Iarm>"
  Demux1/1 -> Iarm_T2/1
  Demux1/2 -> Vmmc_T2/1

== system Controllers/sorting Tmuxed ==
  V1 : Inport
  V2 : Inport  Port=2
  Enable : EnablePort
  Compare To Zero : simulink/Logic and Bit Operations/Compare To Zero  relop===  OutDataTypeStr=uint8
  Counter Limited : simulink/Sources/Counter Limited  uplimit=11  tsamp=Ts
  Demux1 : Demux  Outputs=6
  Demux3 : Demux  Outputs=6
  MATLAB Function VBC1 case 8 : MATLAB Function  TreatAsAtomicUnit=on
  Multiport Switch : MultiPortSwitch  DataPortOrder=Zero-based contiguous  Inputs=12  zeroidx=on  SaturateOnIntegerOverflow=off  InputSameDT=off
  demux : Subsystem
  demux1 : Subsystem
  ind1 : Outport  VectorParamsAs1DForOutWhenUnconnected=off
  ind2 : Outport  Port=2  VectorParamsAs1DForOutWhenUnconnected=off
  wires:
  V1/1 -> Demux1/1
  Counter Limited/1 -> Multiport Switch/1, Compare To Zero/1
  Demux1/1 -> Multiport Switch/2
  Demux1/2 -> Multiport Switch/3
  Demux1/3 -> Multiport Switch/4
  Demux1/4 -> Multiport Switch/5
  Demux1/5 -> Multiport Switch/6
  Demux1/6 -> Multiport Switch/7
  Demux3/1 -> Multiport Switch/8
  Demux3/2 -> Multiport Switch/9
  Demux3/3 -> Multiport Switch/10
  Demux3/4 -> Multiport Switch/11
  Demux3/5 -> Multiport Switch/12
  Demux3/6 -> Multiport Switch/13
  Multiport Switch/1 -> MATLAB Function VBC1 case 8/1(in)
  Compare To Zero/1 -> demux/1(enable)
  MATLAB Function VBC1 case 8/1(ind) -> demux/2(data), demux1/2(data)
  demux/2(endly) -> demux1/1(enable)
  demux/1(do) -> ind1/1
  demux1/1(do) -> ind2/1
  V2/1 -> Demux3/1

== system Controllers/Subsystem/Subsystem1 ==
  In1 : Inport
  CellIndex : Inport  Port=2
  Demux : Demux  Outputs=6
  Mux2 : Mux  Inputs=6
  Subsystem1 : Subsystem
  Subsystem2 : Subsystem
  Subsystem3 : Subsystem
  Subsystem4 : Subsystem
  Subsystem5 : Subsystem
  Subsystem6 : Subsystem
  Vc_SI_to_pu1 : Gain  Gain=1/(E*2/(nb_cell))  SampleTime=Tctrl
  Out1 : Outport  VectorParamsAs1DForOutWhenUnconnected=off
  wires:
  CellIndex/1 -> Subsystem3/2(inx), Subsystem1/2(inx), Subsystem2/2(inx), Subsystem5/2(inx), Subsystem6/2(inx), Subsystem4/2(inx)
  Subsystem6/1(Out1) -> Mux2/6
  Subsystem5/1(Out1) -> Mux2/5
  Subsystem4/1(Out1) -> Mux2/4
  Subsystem2/1(Out1) -> Mux2/3
  In1/1 -> Demux/1
  Subsystem3/1(Out1) -> Mux2/1
  Subsystem1/1(Out1) -> Mux2/2
  Mux2/1 -> Vc_SI_to_pu1/1
  Demux/1 -> Subsystem3/1(In1)
  Demux/2 -> Subsystem1/1(In1)
  Demux/3 -> Subsystem2/1(In1)
  Demux/4 -> Subsystem4/1(In1)
  Demux/5 -> Subsystem5/1(In1)
  Demux/6 -> Subsystem6/1(In1)
  Vc_SI_to_pu1/1 -> Out1/1

== system Controllers/Subsystem/Subsystem3 ==
  In1 : Inport
  Demux : Demux  Outputs=6
  Mux2 : Mux  Inputs=6
  Subsystem1 : Subsystem
  Subsystem2 : Subsystem
  Subsystem3 : Subsystem
  Subsystem4 : Subsystem
  Subsystem5 : Subsystem
  Subsystem6 : Subsystem
  Vc_SI_to_pu1 : Gain  Gain=1/(E*2/(nb_cell/2))  SampleTime=Tctrl
  Out1 : Outport  VectorParamsAs1DForOutWhenUnconnected=off
  wires:
  Vc_SI_to_pu1/1 -> Out1/1
  Demux/6 -> Subsystem5/1(In1)
  Demux/5 -> Subsystem4/1(In1)
  Demux/4 -> Subsystem6/1(In1)
  Demux/3 -> Subsystem2/1(In1)
  Demux/2 -> Subsystem1/1(In1)
  Demux/1 -> Subsystem3/1(In1)
  Mux2/1 -> Vc_SI_to_pu1/1
  Subsystem5/1(Out1) -> Mux2/6
  Subsystem4/1(Out1) -> Mux2/5
  Subsystem6/1(Out1) -> Mux2/4
  Subsystem2/1(Out1) -> Mux2/3
  Subsystem1/1(Out1) -> Mux2/2
  Subsystem3/1(Out1) -> Mux2/1
  In1/1 -> Demux/1

== system Controllers/Subsystem2/Subsystem ==
  In1 : Inport
  Bus Creator : BusCreator  Inputs=6
  Demux3 : Demux  Outputs=[ 6 6 ]
  Subsystem3 : Subsystem
  Subsystem4 : Subsystem
  Out1 : Outport  VectorParamsAs1DForOutWhenUnconnected=off
  wires:
  Subsystem3/2(Iabc_pu) -> Bus Creator/2  "Iabc_pu_T1"
  Bus Creator/1 -> Out1/1
  In1/1 -> Demux3/1
  Subsystem4/3(PQpu) -> Bus Creator/6  "PQ_pu_T2"
  Subsystem4/2(Iabc_pu) -> Bus Creator/5  "Iabc_pu_T2"
  Subsystem4/1("vabc_pu ") -> Bus Creator/4  "Vabc_pu_T2"
  Subsystem3/3(PQpu) -> Bus Creator/3  "PQ_pu_T1"
  Subsystem3/1("vabc_pu ") -> Bus Creator/1  "Vabc_pu_T1"
  Demux3/2 -> Subsystem4/1(vi_ac)
  Demux3/1 -> Subsystem3/1(vi_ac)

== system Controllers/Subsystem2/Subsystem2 ==
  In1 : Inport
  Bus Creator : BusCreator  Inputs=2
  Gain : Gain
  Gain2 : Gain  Gain=0.5
  Subtract : Sum  Inputs=1
  Out1 : Outport  VectorParamsAs1DForOutWhenUnconnected=off
  wires:
  Bus Creator/1 -> Out1/1
  In1/1 -> Gain/1
  Gain2/1 -> Bus Creator/2
  Subtract/1 -> Gain2/1
  Gain/1 -> Bus Creator/1, Subtract/1  "vdc_T1x"

== system Controllers/Subsystem2/Subsystem4 ==
  In1 : Inport
  Bus Creator : BusCreator  Inputs=2
  Gain : Gain
  Gain2 : Gain  Gain=0.5
  Subtract : Sum  Inputs=1
  Out1 : Outport  VectorParamsAs1DForOutWhenUnconnected=off
  wires:
  Gain/1 -> Bus Creator/1, Subtract/1  "vdc_T2x"
  Subtract/1 -> Gain2/1
  Gain2/1 -> Bus Creator/2
  In1/1 -> Gain/1
  Bus Creator/1 -> Out1/1

== system Controllers/VSC controller1/Discrete 2nd-Order Filter ==
  In : Inport
  Discrete State-Space : DiscreteStateSpace  A=Ad  B=Bd  C=Cd  D=Dd  InitialCondition=x0d  SampleTime=Ts
  Out : Outport  InitialOutput=0  VectorParamsAs1DForOutWhenUnconnected=off
  wires:
  In/1 -> Discrete State-Space/1
  Discrete State-Space/1 -> Out/1

== system Controllers/VSC controller1/Vdc ctrl ==
  dcopen : Inport
  Vdc : Inport  Port=2
  Vcap : Inport  Port=3
  Enable : EnablePort  StatesWhenEnabling=reset
  Add4 : Sum  Inputs=1
  Logical Operator1 : Logic  Operator=OR  Inputs=3  AllPortsSameDT=off  OutDataTypeStr=boolean
  Logical Operator2 : Logic  Operator=NOT  AllPortsSameDT=off  OutDataTypeStr=boolean
  Logical Operator3 : Logic  Operator=OR  AllPortsSameDT=off  OutDataTypeStr=boolean
  Unit Delay : UnitDelay  SampleTime=Ts  HasFrameUpgradeWarning=on
  Vac_SI_to_pu1 : Gain  Gain=1/6  SampleTime=Tctrl
  Vdc_ctrler1 : Subsystem
  moded : Subsystem
  vdcmode : Constant  Value=cm
  Pcor_lft : Outport  OutputWhenDisabled=reset  InitialOutput=0  VectorParamsAs1DForOutWhenUnconnected=off
  mode : Outport  Port=2  OutputWhenDisabled=reset  InitialOutput=0  VectorParamsAs1DForOutWhenUnconnected=off
  wires:
  Unit Delay/1 -> Logical Operator3/2
  Vdc/1 -> moded/2(Vdc), Vdc_ctrler1/1(Vcap)
  Vac_SI_to_pu1/1 -> moded/1(Vcap)  "Vcap, lft, right"
  Vdc_ctrler1/1(delP) -> Pcor_lft/1  "Pclft"
  Vcap/1 -> Add4/1
  Add4/1 -> Vac_SI_to_pu1/1
  moded/1(Nmode) -> Logical Operator1/1, Logical Operator2/1
  vdcmode/1 -> Logical Operator1/2
  Logical Operator1/1 -> Vdc_ctrler1/Enable
  dcopen/1 -> Logical Operator1/3
  Logical Operator2/1 -> Logical Operator3/1
  Logical Operator3/1 -> mode/1, Unit Delay/1

== system Controllers/VSC controller1/armVcap ==
  vcap : Inport
  Add{1..6} (6 alike) : Sum  Inputs=1
  Demux4 : Demux  Outputs=ones(6,1)*numberOfCell
  Mux : Mux  Inputs=6
  Vac_SI_to_pu5 : Gain  Gain=1/(E*2)  SampleTime=Tctrl
  vdif : Outport  VectorParamsAs1DForOutWhenUnconnected=off
  wires:
  Vac_SI_to_pu5/1 -> vdif/1  "a1a2b1b2c1c2"
  vcap/1 -> Demux4/1
  Demux4/1 -> Add4/1
  Demux4/2 -> Add1/1
  Demux4/3 -> Add3/1
  Demux4/4 -> Add2/1
  Demux4/5 -> Add6/1
  Demux4/6 -> Add5/1
  Add4/1 -> Mux/1
  Add1/1 -> Mux/2
  Add3/1 -> Mux/3
  Add2/1 -> Mux/4
  Add6/1 -> Mux/5
  Add5/1 -> Mux/6
  Mux/1 -> Vac_SI_to_pu5/1

== system Controllers/VSC controller1/discrete band pass filter1 ==
  In1 : Inport
  Discrete Transfer Fcn : DiscreteTransferFcn  Numerator=numd  Denominator=dend  InitialStates=inistate  SampleTime=Ts
  Out1 : Outport  VectorParamsAs1DForOutWhenUnconnected=off
  wires:
  In1/1 -> Discrete Transfer Fcn/1
  Discrete Transfer Fcn/1 -> Out1/1

== system Controllers/VSC controller1/otherctrl ==
  Vac_ref : Inport
  theda : Inport  Port=2
  Iarm : Inport  Port=3
  mode : Inport  Port=4
  Vcap : Inport  Port=5
  Enable : EnablePort  StatesWhenEnabling=reset
  3to6 : Subsystem
  Lx : Constant  Value=Lxpu*2
  Memory1 : Memory  InheritSampleTime=on
  Ts : Constant  Value=Ts
  VSCController_ctrl : Subsystem
  Vdcref : Constant
  cur-cal : Subsystem
  ver : Constant  Value=2
  xtrIctrl1 : Constant  Value=xtrIctrl1
  zero : Constant  Value=0
  ref : Outport  VectorParamsAs1DForOutWhenUnconnected=off
  wires:
  zero/1 -> VSCController_ctrl/7(P_ref), VSCController_ctrl/6(Idc0)  "vdcref"
  VSCController_ctrl/1(ref) -> ref/1
  Vac_ref/1 -> 3to6/1(In1)  "Vac_ref"
  Vcap/1 -> VSCController_ctrl/3(Vcap)  "Vcap"
  mode/1 -> VSCController_ctrl/4(mode)  "mode"
  Iarm/1 -> cur-cal/1(In1)  "Iarm"
  Vdcref/1 -> VSCController_ctrl/8(vdcref)  "vdcref"
  theda/1 -> VSCController_ctrl/9(theda_eVLP)  "abc"
  ver/1 -> VSCController_ctrl/12(ver)
  VSCController_ctrl/2(hiso) -> Memory1/1
  Memory1/1 -> VSCController_ctrl/2(hisi_VcLP)
  Ts/1 -> VSCController_ctrl/13(Ts)
  xtrIctrl1/1 -> VSCController_ctrl/11(ctrlI)
  cur-cal/1(Out1) -> VSCController_ctrl/5(Iarm)
  3to6/1(Out1) -> VSCController_ctrl/1(Vac_ref)
  Lx/1 -> VSCController_ctrl/10(Lx_ctrl3)

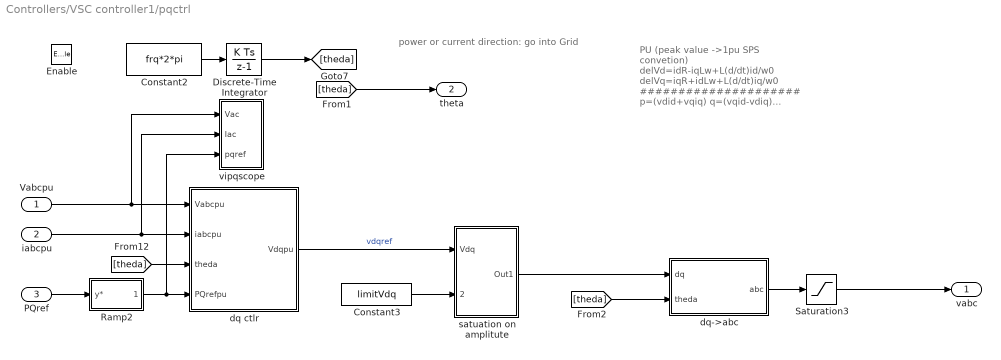
== system Controllers/VSC controller1/pqctrl ==
  note: power or current direction: go into Grid
  note: PU
      | (peak value ->1pu
      | SPS convetion)
      |
      | delVd=idR-iqLw+L(d/dt)id/w0
      | delVq=iqR+idLw+L(d/dt)iq/w0
      | #####################
      | p=(vdid+vqiq)
      | q=(vqid-vdiq)
      | =>
      | Id=(Vd*P+Vq*Q)/C
      | Iq=(Vq*P-Vd*Q)/C
      | C=Vd^2+Vq^2
  Vabcpu : Inport
  iabcpu : Inport  Port=2
  PQref : Inport  Port=3
  Enable : EnablePort  StatesWhenEnabling=reset
  Constant2 : Constant  Value=frq*2*pi
  Constant3 : Constant  Value=limitVdq
  Discrete-Time Integrator : DiscreteIntegrator  SampleTime=Ts  ICPrevOutput=DiscIntNeverNeededParam  ICPrevScaledInput=DiscIntNeverNeededParam
  Ramp2 : Subsystem  mask{ramp=frq/5; %P or Q from 0 to 1pu at 5 cycles}
      mask prompts: ramp "delY/delt"
  Saturation3 : Saturate  UpperLimit=Vabc_lim(2)  LowerLimit=Vabc_lim(1)
  dq ctlr : Subsystem
  dq->abc : Subsystem
  "satuation on amplitute " : Subsystem
  vipqscope : Subsystem
  vabc : Outport  VectorParamsAs1DForOutWhenUnconnected=off
  theta : Outport  Port=2  VectorParamsAs1DForOutWhenUnconnected=off
  wires:
  [theda] -> theta/1
  PQref/1 -> Ramp2/1(y*)
  iabcpu/1 -> dq ctlr/2(iabcpu), vipqscope/2(Iac)
  Vabcpu/1 -> dq ctlr/1(Vabcpu), vipqscope/1(Vac)
  dq ctlr/1(Vdqpu) -> "satuation on amplitute "/1(Vdq)  "vdqref"
  [theda] -> dq ctlr/3(theda)
  Discrete-Time Integrator/1 -> [theda]
  Constant2/1 -> Discrete-Time Integrator/1
  Ramp2/1(yramp*) -> dq ctlr/4(PQrefpu), vipqscope/3(pqref)
  "satuation on amplitute "/1(Out1) -> dq->abc/1(dq)
  Constant3/1 -> "satuation on amplitute "/2(limitVdq)
  dq->abc/1(abc) -> Saturation3/1
  [theda] -> dq->abc/2(theda)
  Saturation3/1 -> vabc/1

== system Controllers/VSC controller2/Discrete 2nd-Order Filter ==
  In : Inport
  Discrete State-Space : DiscreteStateSpace  A=Ad  B=Bd  C=Cd  D=Dd  InitialCondition=x0d  SampleTime=Ts
  Out : Outport  InitialOutput=0  VectorParamsAs1DForOutWhenUnconnected=off
  wires:
  In/1 -> Discrete State-Space/1
  Discrete State-Space/1 -> Out/1

== system Controllers/VSC controller2/Vdc ctrl ==
  dcopen : Inport
  Vdc : Inport  Port=2
  Vcap : Inport  Port=3
  Enable : EnablePort  StatesWhenEnabling=reset
  Add4 : Sum  Inputs=1
  Logical Operator1 : Logic  Operator=OR  Inputs=3  AllPortsSameDT=off  OutDataTypeStr=boolean
  Logical Operator2 : Logic  Operator=NOT  AllPortsSameDT=off  OutDataTypeStr=boolean
  Logical Operator3 : Logic  Operator=OR  AllPortsSameDT=off  OutDataTypeStr=boolean
  Unit Delay : UnitDelay  SampleTime=Ts  HasFrameUpgradeWarning=on
  Vac_SI_to_pu1 : Gain  Gain=1/6  SampleTime=Tctrl
  Vdc_ctrler1 : Subsystem
  moded : Subsystem
  vdcmode : Constant  Value=cm
  Pcor_lft : Outport  OutputWhenDisabled=reset  InitialOutput=0  VectorParamsAs1DForOutWhenUnconnected=off
  mode : Outport  Port=2  OutputWhenDisabled=reset  InitialOutput=0  VectorParamsAs1DForOutWhenUnconnected=off
  wires:
  Unit Delay/1 -> Logical Operator3/2
  Logical Operator3/1 -> mode/1, Unit Delay/1
  Logical Operator2/1 -> Logical Operator3/1
  dcopen/1 -> Logical Operator1/3
  Logical Operator1/1 -> Vdc_ctrler1/Enable
  vdcmode/1 -> Logical Operator1/2
  moded/1(Nmode) -> Logical Operator2/1, Logical Operator1/1
  Add4/1 -> Vac_SI_to_pu1/1
  Vcap/1 -> Add4/1
  Vdc_ctrler1/1(delP) -> Pcor_lft/1  "Pclft"
  Vac_SI_to_pu1/1 -> moded/1(Vcap)  "Vcap, lft, right"
  Vdc/1 -> Vdc_ctrler1/1(Vcap), moded/2(Vdc)

== system Controllers/VSC controller2/armVcap ==
  vcap : Inport
  Add{1..6} (6 alike) : Sum  Inputs=1
  Demux4 : Demux  Outputs=ones(6,1)*numberOfCell
  Mux : Mux  Inputs=6
  Vac_SI_to_pu5 : Gain  Gain=1/(E*2)  SampleTime=Tctrl
  vdif : Outport  VectorParamsAs1DForOutWhenUnconnected=off
  wires:
  Mux/1 -> Vac_SI_to_pu5/1
  Add5/1 -> Mux/6
  Add6/1 -> Mux/5
  Add2/1 -> Mux/4
  Add3/1 -> Mux/3
  Add1/1 -> Mux/2
  Add4/1 -> Mux/1
  Demux4/6 -> Add5/1
  Demux4/5 -> Add6/1
  Demux4/4 -> Add2/1
  Demux4/3 -> Add3/1
  Demux4/2 -> Add1/1
  Demux4/1 -> Add4/1
  vcap/1 -> Demux4/1
  Vac_SI_to_pu5/1 -> vdif/1  "a1a2b1b2c1c2"

== system Controllers/VSC controller2/discrete band pass filter1 ==
  In1 : Inport
  Discrete Transfer Fcn : DiscreteTransferFcn  Numerator=numd  Denominator=dend  InitialStates=inistate  SampleTime=Ts
  Out1 : Outport  VectorParamsAs1DForOutWhenUnconnected=off
  wires:
  Discrete Transfer Fcn/1 -> Out1/1
  In1/1 -> Discrete Transfer Fcn/1

== system Controllers/VSC controller2/otherctrl ==
  Vac_ref : Inport
  theda : Inport  Port=2
  Iarm : Inport  Port=3
  mode : Inport  Port=4
  Vcap : Inport  Port=5
  Enable : EnablePort  StatesWhenEnabling=reset
  3to6 : Subsystem
  Lx : Constant  Value=Lxpu*2
  Memory1 : Memory  InheritSampleTime=on
  Ts : Constant  Value=Ts
  VSCController_ctrl : Subsystem
  Vdcref : Constant
  cur-cal : Subsystem
  xtrIctrl1 : Constant  Value=xtrIctrl1
  zero : Constant  Value=0
  ref : Outport  VectorParamsAs1DForOutWhenUnconnected=off
  wires:
  zero/1 -> VSCController_ctrl/6(Idc0), VSCController_ctrl/7(P_ref)  "vdcref"
  VSCController_ctrl/1(ref) -> ref/1
  Lx/1 -> VSCController_ctrl/10(Lx_ctrl3)
  3to6/1(Out1) -> VSCController_ctrl/1(Vac_ref)
  cur-cal/1(Out1) -> VSCController_ctrl/5(Iarm)
  xtrIctrl1/1 -> VSCController_ctrl/11(ctrlI)
  Ts/1 -> VSCController_ctrl/12(Ts)
  Memory1/1 -> VSCController_ctrl/2(hisi_VcLP)
  VSCController_ctrl/2(hiso) -> Memory1/1
  theda/1 -> VSCController_ctrl/9(theda_eVLP)  "abc"
  Vdcref/1 -> VSCController_ctrl/8(vdcref)  "vdcref"
  Iarm/1 -> cur-cal/1(In1)  "Iarm"
  mode/1 -> VSCController_ctrl/4(mode)  "mode"
  Vcap/1 -> VSCController_ctrl/3(Vcap)  "Vcap"
  Vac_ref/1 -> 3to6/1(In1)  "Vac_ref"

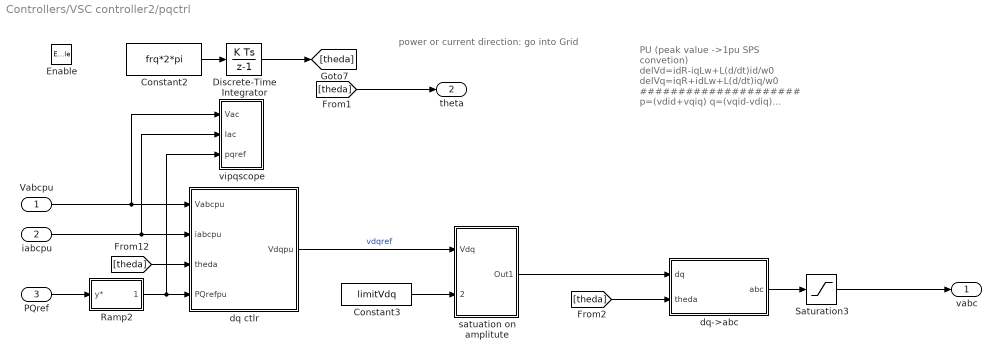
== system Controllers/VSC controller2/pqctrl ==
  note: PU
      | (peak value ->1pu
      | SPS convetion)
      |
      | delVd=idR-iqLw+L(d/dt)id/w0
      | delVq=iqR+idLw+L(d/dt)iq/w0
      | #####################
      | p=(vdid+vqiq)
      | q=(vqid-vdiq)
      | =>
      | Id=(Vd*P+Vq*Q)/C
      | Iq=(Vq*P-Vd*Q)/C
      | C=Vd^2+Vq^2
  note: power or current direction: go into Grid
  Vabcpu : Inport
  iabcpu : Inport  Port=2
  PQref : Inport  Port=3
  Enable : EnablePort  StatesWhenEnabling=reset
  Constant2 : Constant  Value=frq*2*pi
  Constant3 : Constant  Value=limitVdq
  Discrete-Time Integrator : DiscreteIntegrator  SampleTime=Ts  ICPrevOutput=DiscIntNeverNeededParam  ICPrevScaledInput=DiscIntNeverNeededParam
  Ramp2 : Subsystem  mask{ramp=frq/5; %P or Q from 0 to 1pu at 5 cycles}
      mask prompts: ramp "delY/delt"
  Saturation3 : Saturate  UpperLimit=Vabc_lim(2)  LowerLimit=Vabc_lim(1)
  dq ctlr : Subsystem
  dq->abc : Subsystem
  "satuation on amplitute " : Subsystem
  vipqscope : Subsystem
  vabc : Outport  VectorParamsAs1DForOutWhenUnconnected=off
  theta : Outport  Port=2  VectorParamsAs1DForOutWhenUnconnected=off
  wires:
  Saturation3/1 -> vabc/1
  [theda] -> dq->abc/2(theda)
  dq->abc/1(abc) -> Saturation3/1
  Constant3/1 -> "satuation on amplitute "/2(limitVdq)
  "satuation on amplitute "/1(Out1) -> dq->abc/1(dq)
  Ramp2/1(yramp*) -> vipqscope/3(pqref), dq ctlr/4(PQrefpu)
  Constant2/1 -> Discrete-Time Integrator/1
  Discrete-Time Integrator/1 -> [theda]
  [theda] -> dq ctlr/3(theda)
  dq ctlr/1(Vdqpu) -> "satuation on amplitute "/1(Vdq)  "vdqref"
  Vabcpu/1 -> vipqscope/1(Vac), dq ctlr/1(Vabcpu)
  iabcpu/1 -> vipqscope/2(Iac), dq ctlr/2(iabcpu)
  PQref/1 -> Ramp2/1(y*)
  [theda] -> theta/1

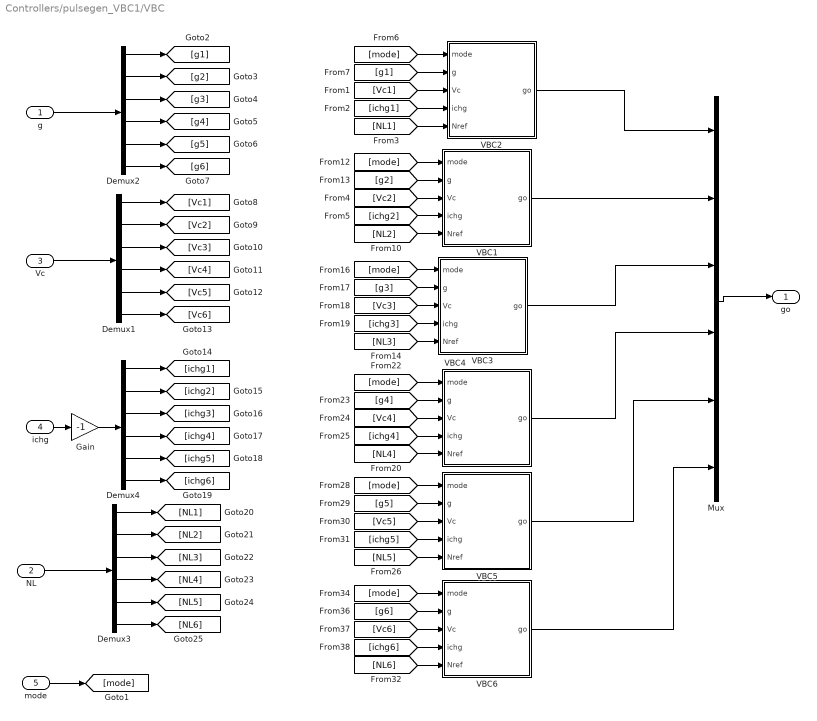
== system Controllers/pulsegen_VBC1/VBC ==
  g : Inport
  NL : Inport  Port=2
  Vc : Inport  Port=3
  ichg : Inport  Port=4
  mode : Inport  Port=5
  Demux{1..4} (4 alike) : Demux  Outputs=6
  Gain : Gain  Gain=-1
  Mux : Mux  Inputs=ones(6,1)*numberOfCell
  VBC1 : Subsystem
  VBC2 : Subsystem
  VBC3 : Subsystem
  VBC4 : Subsystem
  VBC5 : Subsystem
  VBC6 : Subsystem
  go : Outport  VectorParamsAs1DForOutWhenUnconnected=off
  wires:
  VBC2/1(go) -> Mux/1
  Mux/1 -> go/1
  VBC6/1(go) -> Mux/6
  VBC5/1(go) -> Mux/5
  VBC4/1(go) -> Mux/4
  VBC3/1(go) -> Mux/3
  VBC1/1(go) -> Mux/2
  ichg/1 -> Gain/1
  Vc/1 -> Demux1/1
  g/1 -> Demux2/1
  Gain/1 -> Demux4/1
  mode/1 -> [mode]
  [mode] -> VBC2/1(mode)
  Demux2/1 -> [g1]
  Demux2/2 -> [g2]
  Demux2/3 -> [g3]
  Demux2/4 -> [g4]
  Demux2/5 -> [g5]
  Demux2/6 -> [g6]
  [g1] -> VBC2/2(g)
  Demux1/1 -> [Vc1]
  Demux1/2 -> [Vc2]
  Demux1/3 -> [Vc3]
  Demux1/4 -> [Vc4]
  Demux1/5 -> [Vc5]
  Demux1/6 -> [Vc6]
  Demux4/1 -> [ichg1]
  Demux4/2 -> [ichg2]
  Demux4/3 -> [ichg3]
  Demux4/4 -> [ichg4]
  Demux4/5 -> [ichg5]
  Demux4/6 -> [ichg6]
  NL/1 -> Demux3/1
  Demux3/1 -> [NL1]
  Demux3/2 -> [NL2]
  Demux3/3 -> [NL3]
  Demux3/4 -> [NL4]
  Demux3/5 -> [NL5]
  Demux3/6 -> [NL6]
  [Vc1] -> VBC2/3(Vc)
  [ichg1] -> VBC2/4(ichg)
  [NL1] -> VBC2/5(Nref)
  [mode] -> VBC1/1(mode)
  [g2] -> VBC1/2(g)
  [Vc2] -> VBC1/3(Vc)
  [ichg2] -> VBC1/4(ichg)
  [NL2] -> VBC1/5(Nref)
  [mode] -> VBC3/1(mode)
  [g3] -> VBC3/2(g)
  [Vc3] -> VBC3/3(Vc)
  [ichg3] -> VBC3/4(ichg)
  [NL3] -> VBC3/5(Nref)
  [mode] -> VBC4/1(mode)
  [g4] -> VBC4/2(g)
  [Vc4] -> VBC4/3(Vc)
  [ichg4] -> VBC4/4(ichg)
  [NL4] -> VBC4/5(Nref)
  [mode] -> VBC5/1(mode)
  [g5] -> VBC5/2(g)
  [Vc5] -> VBC5/3(Vc)
  [ichg5] -> VBC5/4(ichg)
  [NL5] -> VBC5/5(Nref)
  [mode] -> VBC6/1(mode)
  [g6] -> VBC6/2(g)
  [Vc6] -> VBC6/3(Vc)
  [ichg6] -> VBC6/4(ichg)
  [NL6] -> VBC6/5(Nref)
